simulink model "rtwdemo_param_variants_model"  (Simulink 7.6)
settings: Solver=FixedStepDiscrete  StartTime=0.0  StopTime=10.0  RelTol=1e-3
undefined symbols (not defined in the file or in its folder): Pa1, Pa2, Pb1, Pb2
settings Model: cscVariantNum=2  cscVariantClass1=ECoderDemos.Amplify  cscVariantClass2=ECoderDemos.Bias  Creator=The MathWorks Inc.
settings OptimizationCC: InlineParams=on  UseIntDivNetSlope=on  InlineInvariantSignals=on  EnhancedBackFolding=on  BooleansAsBitfields=on  PassReuseOutputArgsAs=Individual arguments  StateBitsets=on  DataBitsets=on  UseTempVars=on  ZeroExternalMemoryAtStartup=off  ZeroInternalMemoryAtStartup=off  NoFixptDivByZeroProtection=on  EfficientFloat2IntCast=on  OptimizeModelRefInitCode=on  LifeSpan=1
settings DebuggingCC: StrictBusMsg=Warning
settings HardwareCC: ProdBitPerLong=64  ProdIntDivRoundTo=Zero  ProdEndianess=LittleEndian  ProdWordSize=64  ProdHWDeviceType=Specified
settings RTWCC: SystemTargetFile=ert.tlc  TemplateMakefile=ert_default_tmf  Description=Real-Time Workshop Embedded Coder  GenerateReport=on  RTWVerbose=off  ProcessScript=ert_make_rtw_hook  IncludeHyperlinkInReport=on  LaunchReport=on  GenerateTraceInfo=on  GenerateTraceReport=on  GenerateTraceReportSl=on  GenerateTraceReportSf=on  GenerateTraceReportEml=on
settings CodeAppCC: ForceParamTrailComments=on  IgnoreCustomStorageClasses=off  SimulinkDataObjDesc=on  CustomSymbolStrGlobalVar=rt$N$M  CustomSymbolStrType=$N$M  CustomSymbolStrFcn=$N$M$F  CustomSymbolStrMacro=$N$M  InsertBlockDesc=on
settings ERTTargetCC: MultiwordLength=2048  GenerateSampleERTMain=on  IncludeMdlTerminateFcn=off  SupportNonFinite=off  SupportComplex=off  InlinedParameterPlacement=NonHierarchical  ERTCustomFileTemplate=example_file_process.tlc  ERTFilePackagingFormat=CompactWithDataFile  ConvertIfToSwitch=off

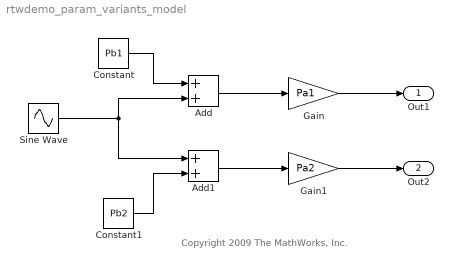
== system rtwdemo_param_variants_model ==
  note: Copyright 2009 The MathWorks, Inc.
  Add : Sum
  Add1 : Sum
  Constant : Constant  Value=Pb1
  Constant1 : Constant  Value=Pb2
  Gain : Gain  Gain=Pa1
  Gain1 : Gain  Gain=Pa2
  Sine Wave : Sin  SineType=Sample based  Frequency=20  Samples=20  SampleTime=0.1
  Out1 : Outport
  Out2 : Outport  Port=2
  wires:
  Constant/1 -> Add/1
  Sine Wave/1 -> Add/2, Add1/1
  Constant1/1 -> Add1/2
  Add/1 -> Gain/1
  Add1/1 -> Gain1/1
  Gain1/1 -> Out2/1
  Gain/1 -> Out1/1
